simulink model "UserOneButton"  (R2019b)
settings: Solver=FixedStepAuto  StartTime=0.0  StopTime=10.0  RelTol=1e-3
undefined symbols (not defined in the file): PWMPeriod_D
libraries: simulink x2
settings Model: DataDictionary=UserOneButtonInterface.sldd  OrderedModelArguments=off  Creator=unix  LastModifiedBy=unix

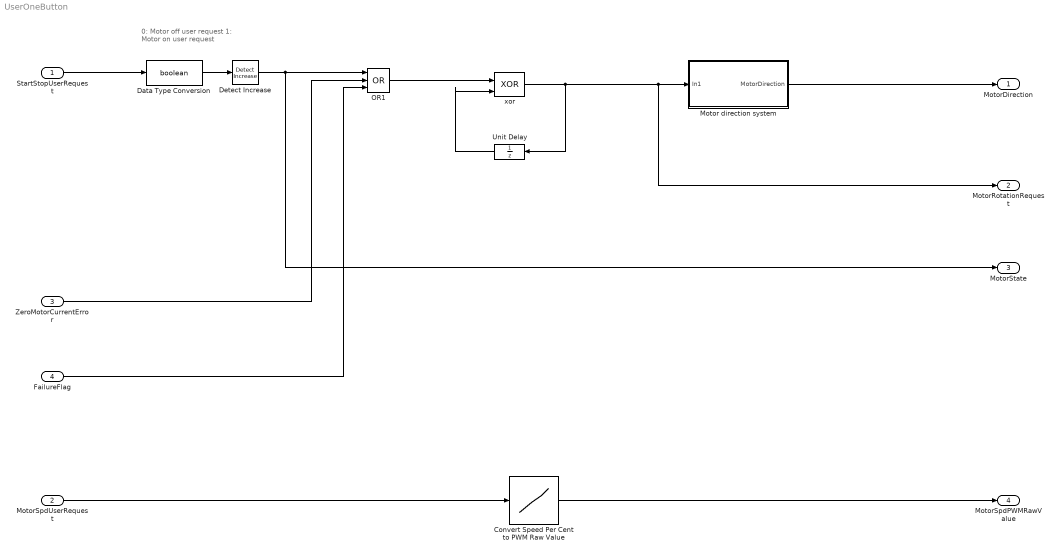
== system UserOneButton ==
  note: 0: Motor off user request
      | 1: Motor on user request
  StartStopUserRequest : Inport  OutDataTypeStr=Enum: MotorStates_e
  MotorSpdUserRequest : Inport  Port=2  OutDataTypeStr=uint8
  ZeroMotorCurrentError : Inport  Port=3
  FailureFlag : Inport  Port=4
  Convert Speed Per Cent to PWM Raw Value : Lookup_n-D  NumberOfTableDimensions=1  BreakpointsForDimension1=[0 100]  Table=[0 PWMPeriod_D]  ExtrapMethod=Clip  InternalRulePriority=Speed  OutDataTypeStr=Inherit: Inherit from 'Table data'  RndMeth=Simplest  InputSameDT=on
  Data Type Conversion : DataTypeConversion  OutDataTypeStr=boolean
  Detect Increase : simulink/Logic and Bit Operations/Detect Increase  vinit=0.0  OutDataTypeStr=boolean
  Motor direction system : Subsystem
  OR1 : Logic  Operator=OR  Inputs=3  IconShape=distinctive  AllPortsSameDT=off  OutDataTypeStr=boolean
  Unit Delay : UnitDelay  SampleTime=-1  HasFrameUpgradeWarning=on
  "xor " : Logic  Operator=XOR  IconShape=distinctive  AllPortsSameDT=off  OutDataTypeStr=boolean
  MotorDirection : Outport
  MotorRotationRequest : Outport  Port=2
  MotorState : Outport  Port=3
  MotorSpdPWMRawValue : Outport  Port=4
  wires:
  ZeroMotorCurrentError/1 -> OR1/2
  StartStopUserRequest/1 -> Data Type Conversion/1
  MotorSpdUserRequest/1 -> Convert Speed Per Cent to PWM Raw Value/1
  "xor "/1 -> MotorRotationRequest/1, Motor direction system/1(In1), Unit Delay/1
  Unit Delay/1 -> "xor "/2
  Motor direction system/1(MotorDirection) -> MotorDirection/1
  Detect Increase/1 -> MotorState/1, OR1/1
  OR1/1 -> "xor "/1
  FailureFlag/1 -> OR1/3
  Data Type Conversion/1 -> Detect Increase/1
  Convert Speed Per Cent to PWM Raw Value/1 -> MotorSpdPWMRawValue/1

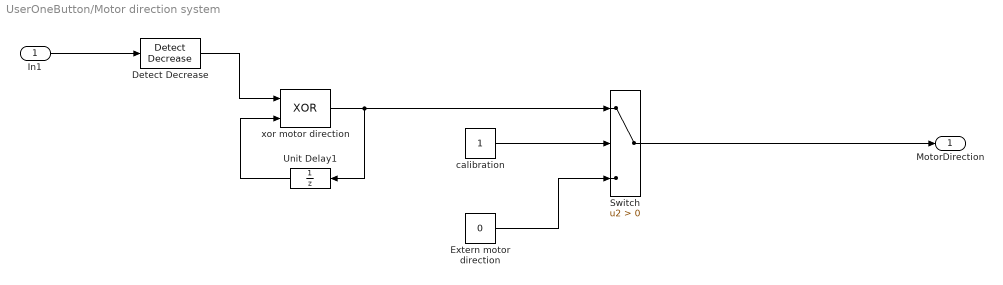
== system UserOneButton/Motor direction system ==
  In1 : Inport
  Detect Decrease : simulink/Logic and Bit Operations/Detect Decrease  vinit=0.0  OutDataTypeStr=boolean
  Extern motor direction : Constant  Value=0  OutDataTypeStr=boolean
  Switch : Switch  Criteria=u2 > Threshold
  Unit Delay1 : UnitDelay  SampleTime=-1  HasFrameUpgradeWarning=on
  "calibration " : Constant  OutDataTypeStr=boolean
  xor motor direction : Logic  Operator=XOR  IconShape=distinctive  AllPortsSameDT=off  OutDataTypeStr=boolean
  MotorDirection : Outport  VectorParamsAs1DForOutWhenUnconnected=off
  wires:
  Unit Delay1/1 -> xor motor direction/2
  In1/1 -> Detect Decrease/1
  Switch/1 -> MotorDirection/1
  Detect Decrease/1 -> xor motor direction/1
  xor motor direction/1 -> Unit Delay1/1, Switch/1
  Extern motor direction/1 -> Switch/3
  "calibration "/1 -> Switch/2
